simulink model "resistance"  (Simulink 7.4)
settings: Solver=ode45  StartTime=0.0  StopTime=10.0  RelTol=1e-3
settings Model: Creator=Administrator  LastModifiedBy=Administrator

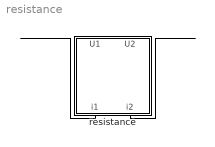
== system resistance ==
  resistance : Subsystem
  wires:
  ? -> resistance/1(U1)
  resistance/1(i1) -> ?
  resistance/2(i2) -> ?
  ? -> resistance/2(U2)

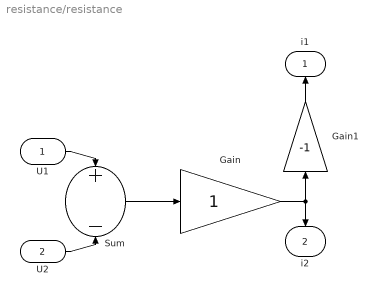
== system resistance/resistance ==
  U1 : Inport
  U2 : Inport  Port=2
  Gain : Gain  ParameterDataType=fixdt(1, 16)  ParameterScaling=2^0  OutDataType=fixdt(1, 16)  OutScaling=2^0
  Gain1 : Gain  Gain=-1  ParameterDataType=fixdt(1, 16)  ParameterScaling=2^0  OutDataType=fixdt(1, 16)  OutScaling=2^0
  Sum : Sum  Inputs=+|-  OutDataType=fixdt(1, 16)  OutScaling=2^0
  i1 : Outport
  i2 : Outport  Port=2
  wires:
  Sum/1 -> Gain/1
  Gain/1 -> Gain1/1, i2/1
  Gain1/1 -> i1/1
  U1/1 -> Sum/1
  U2/1 -> Sum/2
